simulink model "combind5lvl12"  (Simulink 7.3)
settings: Solver=ode45  StartTime=0.0  StopTime=1  RelTol=1e-3
libraries: powerlib x14, simulink x5
settings Model: Creator=DILEEP KUMAR  LastModifiedBy=ayyapa
settings DebuggingCC: FcnCallInpInsideContextMsg=Enable All  StrictBusMsg=ErrorLevel1
settings GRTTargetCC: CombineOutputUpdateFcns=on

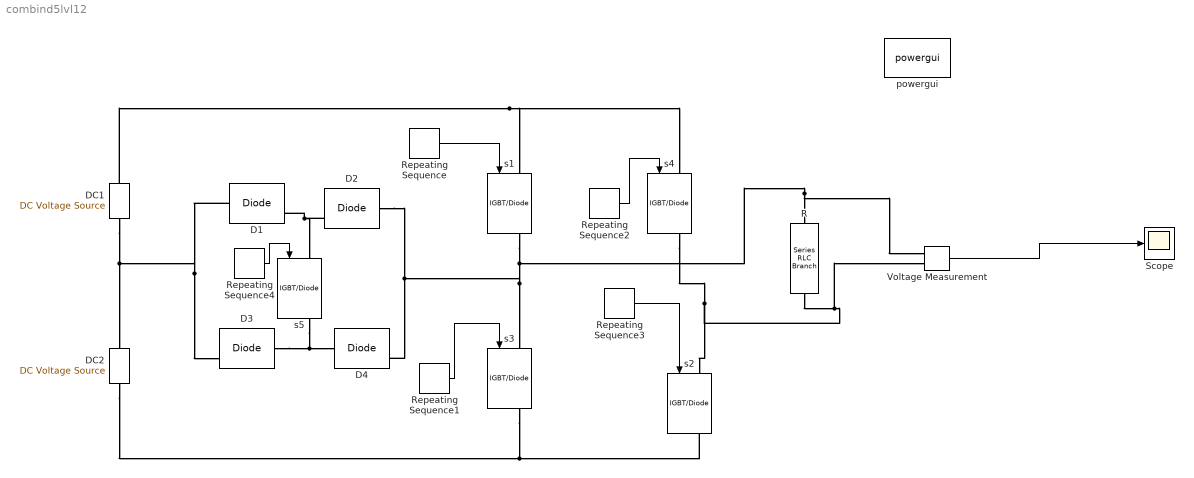
== system combind5lvl12 ==
  " R" : powerlib/Elements/Series RLC Branch  DialogController=POWERSYS.PowerSysDialog  PhysicalDomain=powersysdomain  SubClassName=unknown  LeftPortType=p1  RightPortType=p1  LConnTagsString=__new0  RConnTagsString=__new0  BranchType=R  Resistance=10  Inductance=1e-3  SetiL0=off  InitialCurrent=0  Capacitance=1e-6  Setx0=off  InitialVoltage=0  Measurements=None
  D{1..4} (4 alike) : powerlib/Power Electronics/Diode  DialogController=POWERSYS.PowerSysDialog  SystemSampleTime=-1  Ron=0.001  Lon=0  Vf=0.8  IC=0  UseSnubber=off  Rs=500  Cs=250e-9  Measurements=on
  DC1 : powerlib/Electrical Sources/DC Voltage Source  DialogController=POWERSYS.PowerSysDialog  SystemSampleTime=-1  Amplitude=100  Measurements=None
  DC2 : powerlib/Electrical Sources/DC Voltage Source  DialogController=POWERSYS.PowerSysDialog  SystemSampleTime=-1  Amplitude=100  Measurements=None
  Repeating Sequence : simulink/Sources/Repeating Sequence  SystemSampleTime=-1  rep_seq_t=[0 2 2 4 4 10]*(0.02/10)  rep_seq_y=[0 0 1 1 0 0]
  Repeating Sequence1 : simulink/Sources/Repeating Sequence  SystemSampleTime=-1  rep_seq_t=[0 0 1 1 5 5 6 6 7 7 9 9 10]*(0.02/10)  rep_seq_y=[0 1 1 0 0 1 1 0 0 1 1 0 0]
  Repeating Sequence2 : simulink/Sources/Repeating Sequence  SystemSampleTime=-1  rep_seq_t=[0 6 6 10 10]*(0.02/10)  rep_seq_y=[0 0 1 1 0]
  Repeating Sequence3 : simulink/Sources/Repeating Sequence  SystemSampleTime=-1  rep_seq_t=[0 0 6 6 10]*(0.02/10)  rep_seq_y=[0 1 1 0 0]
  Repeating Sequence4 : simulink/Sources/Repeating Sequence  SystemSampleTime=-1  rep_seq_t=[0 1 1 2 2 4 4 5 5 6 6 7 7 9 9 10 10]*(0.02/10)  rep_seq_y=[0 0 1 1 0 0 1 1 0 0 1 1 0 0 1 1 0]
  Scope : Scope
      settings: SaveName=combinedh
  Voltage Measurement : powerlib/Measurements/Voltage Measurement  DialogController=POWERSYS.PowerSysDialog  SystemSampleTime=-1  PhasorSimulation=off  OutputType=Complex  PSBequivalent=0
  powergui : powerlib/powergui  Priority=1  SystemSampleTime=-1  SimulationMode=Continuous  SampleTime=50e-6  frequency=60  SPID=off  DisableSnubberDevices=off  DisableRonSwitches=off  DisableVfSwitches=off  SwTol=0  Interpol=off  frequencyindice=0  echomessages=off  HookPort=off  DisplayEquations=off  FunctionMessages=off  EnableUseOfTLC=off  x0status=blocks  RestoreLinks=warning  Frange=[0:2:500]  Ylog=off  Xlog=on  ShowGrid=off  save=off  variable=ZData  structure=combinedh  ZoomFFT=off  StartTime=0.2  cycles=1  DisplayStyle=1  fundamental=50  FreqAxis=off  MaxFrequency=1000  frequencyindicesteady=1  RmsSteady=1  display=off  Ts=0  methode=off
  s{1..5} (5 alike) : powerlib/Power Electronics/IGBT//Diode  DialogController=POWERSYS.PowerSysDialog  SystemSampleTime=-1  Ron=1e-3  Rs=1e5  Cs=inf  Measurements=on
  wires:
  Repeating Sequence1/1 -> s3/1
  Repeating Sequence3/1 -> s2/1
  Repeating Sequence2/1 -> s4/1
  Repeating Sequence/1 -> s1/1
  Voltage Measurement/1 -> Scope/1
  Repeating Sequence4/1 -> s5/1
  connections:
  DC1/LConn1 -- DC2/RConn1 -- D1/LConn1 -- D3/RConn1
  DC2/LConn1 -- s2/RConn1 -- s3/RConn1
  DC1/RConn1 -- s4/LConn1 -- s1/LConn1
  " R"/RConn1 -- s4/RConn1 -- s2/LConn1 -- Voltage Measurement/LConn2
  D2/RConn1 -- D1/RConn1 -- s5/LConn1
  D3/LConn1 -- D4/LConn1 -- s5/RConn1
  s1/RConn1 -- s3/LConn1 -- D2/LConn1 -- D4/RConn1 -- " R"/LConn1 -- Voltage Measurement/LConn1
